simulink model "Cannon_Fire"  (R2019b)
settings: Solver=VariableStepAuto  StartTime=0.0  StopTime=25  RelTol=1e-4
libraries: simulink x1
settings Model: Creator=bala4krish  LastModifiedBy=bala4krish

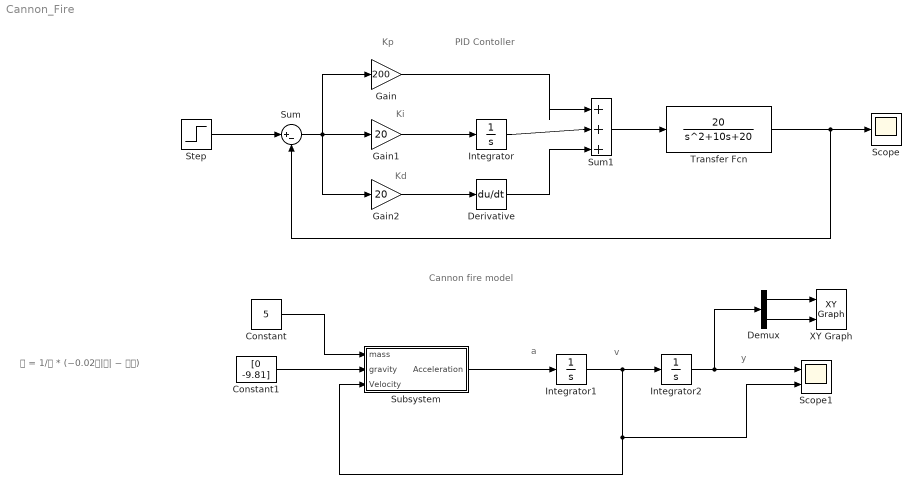
== system Cannon_Fire ==
  note: y
  note: v
  note: a
  note: PID Contoller
  note: 𝑎 = 1/𝑚 * (−0.02𝑣|𝑣| − 𝑚𝑔)
  note: Cannon fire model
  note: Kd
  note: Ki
  note: Kp
  Constant : Constant  Value=5
  Constant1 : Constant  Value=[0 -9.81]
  Demux : Demux  Outputs=2
  Derivative : Derivative
  Gain : Gain  Gain=200
  Gain1 : Gain  Gain=20
  Gain2 : Gain  Gain=20
  Integrator : Integrator
  Integrator1 : Integrator  InitialCondition=[100 100]
  Integrator2 : Integrator  InitialCondition=[0 0]
  Scope : Scope
  Scope1 : Scope  NumInputPorts=2
  Step : Step  Time=0  SampleTime=0
  Subsystem : Subsystem
  Sum : Sum  Inputs=|+-
  Sum1 : Sum  Inputs=|+++
  Transfer Fcn : TransferFcn  Numerator=[20]  Denominator=[1 10 20]
  XY Graph : simulink/Sinks/XY Graph  xmin=0  xmax=500  ymin=0  ymax=250  st=-1
  wires:
  Step/1 -> Sum/1
  Sum/1 -> Gain2/1, Gain/1, Gain1/1
  Gain1/1 -> Integrator/1
  Sum1/1 -> Transfer Fcn/1
  Integrator/1 -> Sum1/2
  Gain/1 -> Sum1/1
  Gain2/1 -> Derivative/1
  Derivative/1 -> Sum1/3
  Transfer Fcn/1 -> Sum/2, Scope/1
  Constant/1 -> Subsystem/1(mass)
  Constant1/1 -> Subsystem/2(gravity)
  Subsystem/1(Acceleration) -> Integrator1/1
  Integrator1/1 -> Scope1/2, Subsystem/3(Velocity), Integrator2/1
  Integrator2/1 -> Demux/1, Scope1/1
  Demux/1 -> XY Graph/1
  Demux/2 -> XY Graph/2

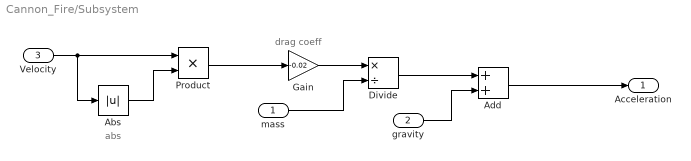
== system Cannon_Fire/Subsystem ==
  note: drag coeff
  note: abs
  mass : Inport
  gravity : Inport  Port=2
  Velocity : Inport  Port=3
  Abs : Abs
  Add : Sum
  Divide : Product  Inputs=*/
  Gain : Gain  Gain=-0.02
  Product : Product
  Acceleration : Outport
  wires:
  Velocity/1 -> Abs/1, Product/1
  Abs/1 -> Product/2
  Product/1 -> Gain/1
  Gain/1 -> Divide/1
  mass/1 -> Divide/2
  Divide/1 -> Add/1
  Add/1 -> Acceleration/1
  gravity/1 -> Add/2
